simulink model "TradeStudyBattery"  (R2024a)
settings: Solver=FixedStepDiscrete  StartTime=0.0  StopTime=10  RelTol=1e-3  EnableMultiTasking=on
PreLoadFcn:
  | V = 0;
InitFcn:
  | V = str2double(get_param('TradeStudyBattery/Trade Study Options','Value'));
settings Model: Creator=callie  LastModifiedBy=callie
settings SolverCC: AutoInsertRateTranBlk=on
settings DataIOCC: SaveOutput=off  SaveTime=off  ReturnWorkspaceOutputs=off
settings OptimizationCC: DefaultParameterBehavior=Inlined  InlineInvariantSignals=on  EnhancedBackFolding=on  PassReuseOutputArgsAs=Individual arguments  StateBitsets=on  DataBitsets=on  ZeroExternalMemoryAtStartup=off  ZeroInternalMemoryAtStartup=off  NoFixptDivByZeroProtection=on  LifeSpan=1  OptimizeBlockOrder=speed  DifferentSizesBufferReuse=on  EfficientTunableParamExpr=on
settings DebuggingCC: ParameterTunabilityLossMsg=error
settings HardwareCC: ProdBitPerPointer=32  ProdBitPerSizeT=32  ProdBitPerPtrDiffT=32  ProdLargestAtomicFloat=None  ProdIntDivRoundTo=Floor  ProdWordSize=32  ProdHWDeviceType=Generic->Custom
settings SFSimCC: MATLABDynamicMemAlloc=off
settings RTWCC: Description=Embedded Coder  SystemTargetFile=ert.tlc  TLCOptions=-p0  GenCodeOnly=on  TemplateMakefile=ert_default_tmf  GenerateReport=on  RTWVerbose=off  IncludeHyperlinkInReport=on  LaunchReport=on
settings CodeAppCC: ForceParamTrailComments=on  IgnoreCustomStorageClasses=off  OperatorAnnotations=on  SimulinkDataObjDesc=on  SFDataObjDesc=on  CustomSymbolStrGlobalVar=rt$N$M  CustomSymbolStrType=$N$M  CustomSymbolStrFcn=$N$M$F  CustomSymbolStrMacro=$N$M  InsertBlockDesc=on
settings ERTTargetCC: TargetLangStandard=C99 (ISO)  CodeReplacementLibrary=ISO_C  GenerateSampleERTMain=on  IncludeMdlTerminateFcn=off  SuppressErrorStatus=on  SupportAbsoluteTime=off  PurelyIntegerCode=on  SupportNonFinite=off  SupportComplex=off  InlinedParameterPlacement=NonHierarchical  RootIOFormat=Structure reference  ERTCustomFileTemplate=example_file_process.tlc

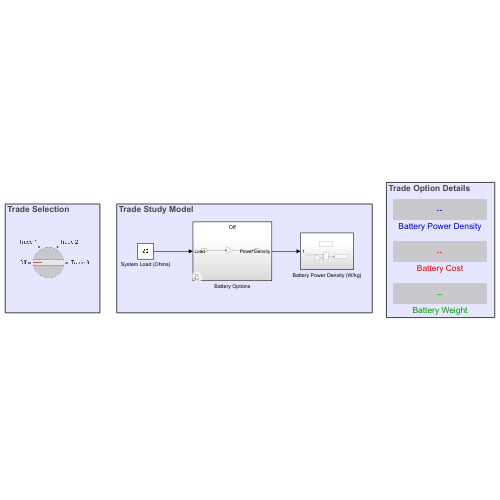
[thumbnail: Simulink's stored preview of the top-level diagram]
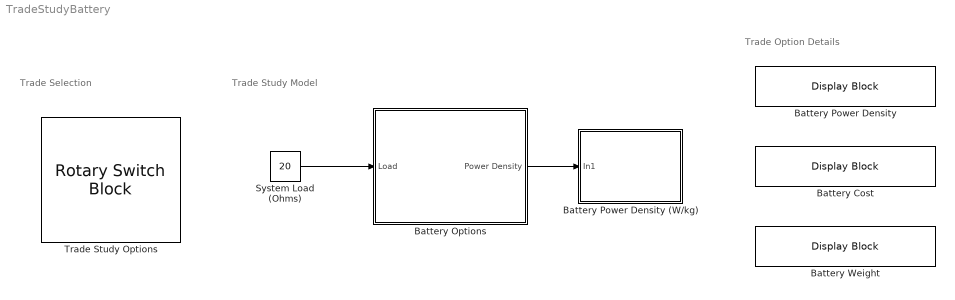
== system TradeStudyBattery ==
  note: Trade Selection
  note: Trade Study Model
  note: Trade Option Details
  Battery Cost : DisplayBlock  LabelPosition=Hide  Format=Custom  Transparency=1  FormatString=$%.2f
  Battery Options : Subsystem  Variant=on  AllowZeroVariantControls=on
  Battery Power Density : DisplayBlock  LabelPosition=Hide  Format=Custom  Transparency=1  FormatString=%.1f W/kg
  Battery Power Density (W/kg) : Subsystem
  Battery Weight : DisplayBlock  LabelPosition=Hide  Format=Custom  Transparency=1  FormatString=%.1f kg
  System Load (Ohms) : Constant  Value=20
  Trade Study Options : RotarySwitchBlock  LabelPosition=Hide
      settings: Values={{'Off', 'Trade 1', 'Trade 2', 'Trade 3'}, [0 1 2 3]}
  wires:
  System Load (Ohms)/1 -> Battery Options/1(Load)
  Battery Options/1(Power Density) -> Battery Power Density (W/kg)/1(In1)

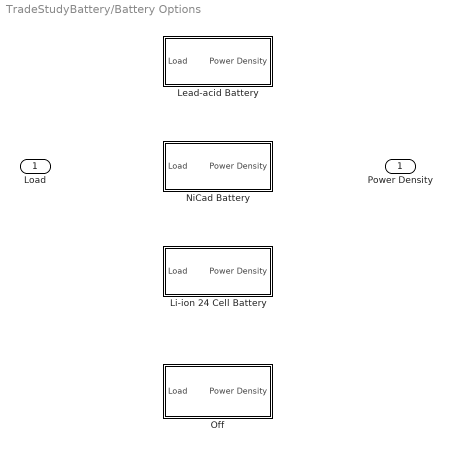
== system TradeStudyBattery/Battery Options ==
  Load : Inport
  Lead-acid Battery : Subsystem  VariantControl=V == 1
  Li-ion 24 Cell Battery : Subsystem  VariantControl=V == 3
  NiCad Battery : Subsystem  VariantControl=V == 2
  Off : Subsystem  VariantControl=V == 0
  Power Density : Outport

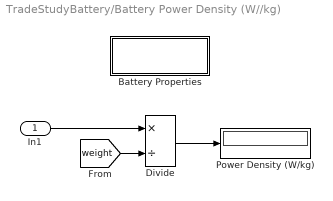
== system TradeStudyBattery/Battery Power Density (W//kg) ==
  In1 : Inport
  Battery Properties : Subsystem
  Divide : Product  Inputs=*/
  Power Density (W/kg) : Display
  wires:
  Divide/1 -> Power Density (W/kg)/1
  In1/1 -> Divide/1
  [weight] -> Divide/2

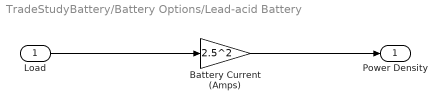
== system TradeStudyBattery/Battery Options/Lead-acid Battery ==
  Load : Inport
  Battery Current (Amps) : Gain  Gain=2.5^2
  Power Density : Outport
  wires:
  Load/1 -> Battery Current (Amps)/1
  Battery Current (Amps)/1 -> Power Density/1

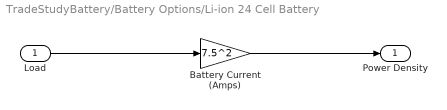
== system TradeStudyBattery/Battery Options/Li-ion 24 Cell Battery ==
  Load : Inport
  Battery Current (Amps) : Gain  Gain=7.5^2
  Power Density : Outport
  wires:
  Load/1 -> Battery Current (Amps)/1
  Battery Current (Amps)/1 -> Power Density/1

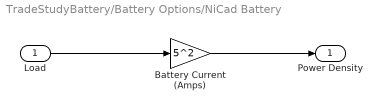
== system TradeStudyBattery/Battery Options/NiCad Battery ==
  Load : Inport
  Battery Current (Amps) : Gain  Gain=5^2
  Power Density : Outport
  wires:
  Load/1 -> Battery Current (Amps)/1
  Battery Current (Amps)/1 -> Power Density/1

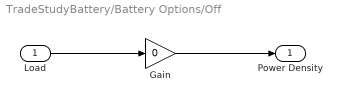
== system TradeStudyBattery/Battery Options/Off ==
  Load : Inport
  Gain : Gain  Gain=0
  Power Density : Outport
  wires:
  Gain/1 -> Power Density/1
  Load/1 -> Gain/1

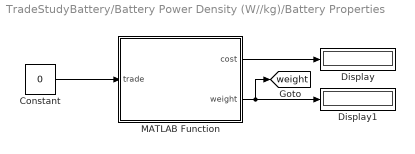
== system TradeStudyBattery/Battery Power Density (W//kg)/Battery Properties ==
  Constant : Constant  Value=0
  Display : Display
  Display1 : Display
      settings: Format=bank
  MATLAB Function : MATLAB Function  TreatAsAtomicUnit=on
  tag scope: weight=global
  wires:
  Constant/1 -> MATLAB Function/1(trade)
  MATLAB Function/1(cost) -> Display/1
  MATLAB Function/2(weight) -> Display1/1, [weight]

== matlab function TradeStudyBattery/Battery Power Density (W//kg)/Battery Properties/MATLAB Function ==
  data: trade input; cost output; weight output
function [cost,weight] = propfcn(trade)

if trade == 1 % Lead-Acid
 cost = 100;
 weight = 0.5;
elseif trade == 2 % NiCad
 cost = 200;
 weight = 1;
elseif trade == 3 % Li-Ion
 cost = 300;
 weight = 2;
else % trade == 0 % Off
 cost = 0;
 weight = 0.001;
end
